simulink model "StraddleCarrier"  (R2022b)
settings: Solver=FixedStepAuto  StartTime=0  StopTime=1000  FixedStep=Ts  RelTol=1e-3
undefined symbols (not defined in the file): AEB, driving, m, n, q, theta, Ts
libraries: simulink x6, roadrunnerscenario x4, simulink_extras x4, drivingscenarioandsensors x3, uavsim3dlib x3, sim3dprobsensorlib x2, trackingutilitieslib x1, drivinglib x1, sim3dlib x1, sim3dcameralib x1, sim3dphyssensorlib x1, sim3dgroundtruthsensorlib x1
(part 2 of 3)

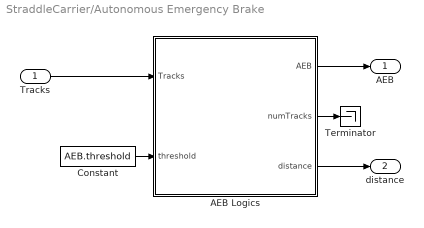
== system StraddleCarrier/Autonomous Emergency Brake ==
  Tracks : Inport  OutDataTypeStr=Bus: BusMultiObjectTracker1  SampleTime=[Ts, 0]  BusOutputAsStruct=on
  AEB Logics : MATLAB Function  TreatAsAtomicUnit=on
  Constant : Constant  Value=AEB.threshold
  Terminator : Terminator
  AEB : Outport  OutDataTypeStr=boolean
  distance : Outport  Port=2
  wires:
  Tracks/1 -> AEB Logics/1(Tracks)
  AEB Logics/1(AEB) -> AEB/1
  Constant/1 -> AEB Logics/2(threshold)
  AEB Logics/3(distance) -> distance/1
  AEB Logics/2(numTracks) -> Terminator/1

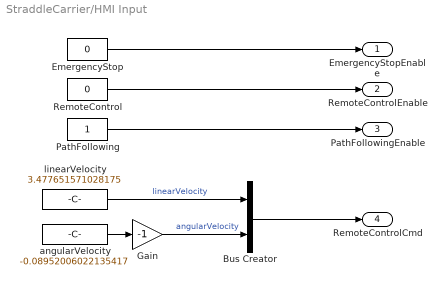
== system StraddleCarrier/HMI Input ==
  Bus Creator : BusCreator  Inputs=2  OutDataTypeStr=Bus: RemoteControlCmd
  EmergencyStop : Constant  Value=0  OutDataTypeStr=boolean
  Gain : Gain  Gain=-1
  PathFollowing : Constant  OutDataTypeStr=boolean
  RemoteControl : Constant  Value=0  OutDataTypeStr=boolean
  angularVelocity : Constant  Value=-0.08952006022135417
  linearVelocity : Constant  Value=3.477651571028175
  EmergencyStopEnable : Outport
  RemoteControlEnable : Outport  Port=2
  PathFollowingEnable : Outport  Port=3
  RemoteControlCmd : Outport  Port=4
  wires:
  RemoteControl/1 -> RemoteControlEnable/1
  linearVelocity/1 -> Bus Creator/1  "linearVelocity"
  PathFollowing/1 -> PathFollowingEnable/1
  angularVelocity/1 -> Gain/1
  EmergencyStop/1 -> EmergencyStopEnable/1
  Bus Creator/1 -> RemoteControlCmd/1
  Gain/1 -> Bus Creator/2  "angularVelocity"

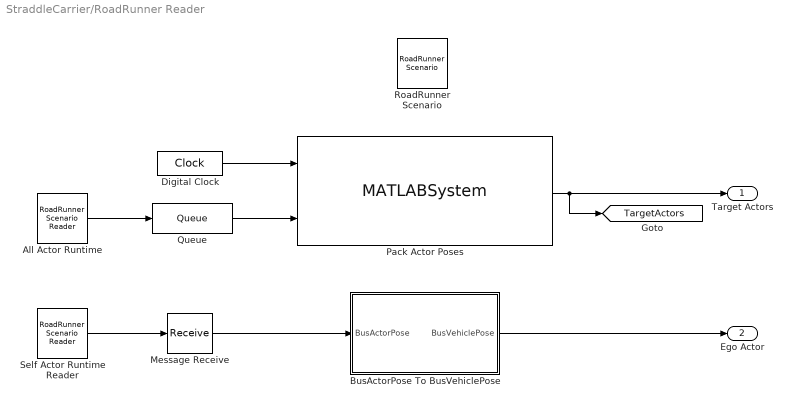
== system StraddleCarrier/RoadRunner Reader ==
  All Actor Runtime : roadrunnerscenario/RoadRunner Scenario Reader  TopicCategory=Actor  ActorCategory=All Types  ActionType=Path Following  TopicType=Actor Pose (Driving Scenario compatible)  VehicleType=Vehicle Specifications  UserDefinedAction=Action1  Filter=None  SampleTime=Ts
  BusActorPose To BusVehiclePose : Subsystem
  Digital Clock : DigitalClock  SampleTime=Ts
  Message Receive : Receive  InputPortMessageModes=m  SampleTime=Ts
  Pack Actor Poses : MATLABSystem  InputPortMessageModes=n,m  System=HelperPackDrivingScenarioPoses  EgoActorID=1  ActorProfiles=struct( 'ActorID', 1, 'ClassID', 1, 'Length', 4.7, 'Width', 1.8, 'Height', 1.4, 'OriginOffset', [ 0, 0, 0 ], 'FrontOverhang', 0, 'RearOverhang', 0, 'Wheelbase', 0, 'Color', [ 0, 0, 0 ] )  DefaultActorPoses="Simulink.Bus.createMATLABStruct( \"BusActors\" )"
      mask Type: HelperPackDrivingScenarioPoses
      mask Display:
      | disp(['HelperPack' char(10) 'DrivingScenarioPoses']);
      | port_label('input',1,'time');
      | port_label('input',2,'msgs');
      | port_label('output',1,'TargetPoses');
  Queue : Queue  InputPortMessageModes=m  OutputPortMessageModes=m  OverwriteOldest=on  Capacity=numActors
  RoadRunner Scenario : roadrunnerscenario/RoadRunner Scenario  UserDefinedActions={}
  Self Actor Runtime Reader : roadrunnerscenario/RoadRunner Scenario Reader  TopicCategory=Actor  ActorCategory=All Types  ActionType=Path Following  TopicType=Actor Pose (Driving Scenario compatible)  VehicleType=Vehicle Specifications  UserDefinedAction=Action1  Filter=Self  SampleTime=Ts
  Target Actors : Outport
  Ego Actor : Outport  Port=2
  tag scope: TargetActors=global
  wires:
  All Actor Runtime/1 -> Queue/1
  Self Actor Runtime Reader/1 -> Message Receive/1
  Queue/1 -> Pack Actor Poses/2
  Pack Actor Poses/1 -> [TargetActors], Target Actors/1
  Message Receive/1 -> BusActorPose To BusVehiclePose/1(BusActorPose)
  BusActorPose To BusVehiclePose/1(BusVehiclePose) -> Ego Actor/1
  Digital Clock/1 -> Pack Actor Poses/1

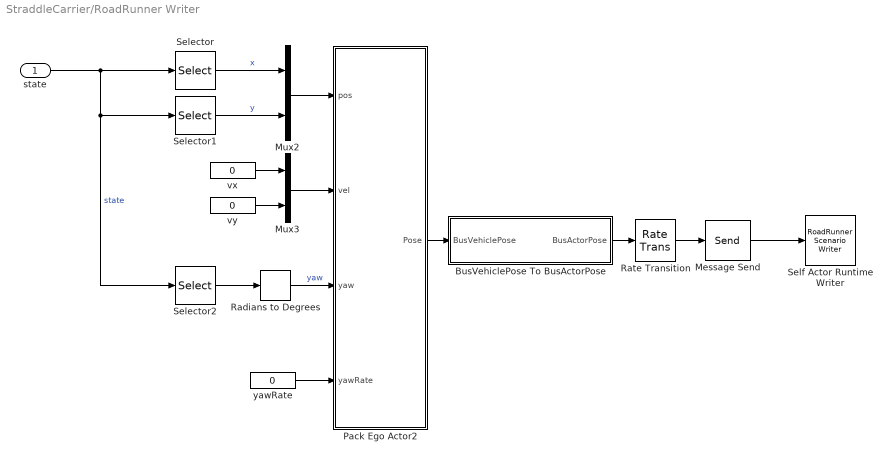
== system StraddleCarrier/RoadRunner Writer ==
  state : Inport
  BusVehiclePose To BusActorPose : Subsystem
  Message Send : Send  OutputPortMessageModes=m
  Mux2 : Mux  Inputs=2
  Mux3 : Mux  Inputs=2
  Pack Ego Actor2 : MATLAB Function  TreatAsAtomicUnit=on  mask{egoActorID=1}
      mask prompts: egoActorID "Ego Actor ID"
  Radians to Degrees : simulink_extras/Transformations/Radians to Degrees
  Rate Transition : RateTransition  OutPortSampleTime=Ts
  Selector : Selector  InputPortWidth=3  IndexOptions=Index vector (dialog)  Indices=[1]  OutputSizes=1
  Selector1 : Selector  InputPortWidth=3  IndexOptions=Index vector (dialog)  Indices=[2]  OutputSizes=1
  Selector2 : Selector  InputPortWidth=3  IndexOptions=Index vector (dialog)  Indices=[3]  OutputSizes=1
  Self Actor Runtime Writer : roadrunnerscenario/RoadRunner Scenario Writer  TopicCategory=Actor  ActorCategory=All Types  EventType=Action Complete  VehicleType=Vehicle Pose  TopicType=Actor Pose (Driving Scenario compatible)
  vx : Constant  Value=0
  vy : Constant  Value=0
  yawRate : Constant  Value=0
  wires:
  BusVehiclePose To BusActorPose/1(BusActorPose) -> Rate Transition/1
  Pack Ego Actor2/1(Pose) -> BusVehiclePose To BusActorPose/1(BusVehiclePose)
  Message Send/1 -> Self Actor Runtime Writer/1
  Rate Transition/1 -> Message Send/1
  Radians to Degrees/1 -> Pack Ego Actor2/3(yaw)  "yaw"
  state/1 -> Selector2/1, Selector1/1, Selector/1  "state"
  vx/1 -> Mux3/1
  vy/1 -> Mux3/2
  Selector1/1 -> Mux2/2  "y"
  Mux3/1 -> Pack Ego Actor2/2(vel)
  Mux2/1 -> Pack Ego Actor2/1(pos)
  Selector/1 -> Mux2/1  "x"
  yawRate/1 -> Pack Ego Actor2/4(yawRate)
  Selector2/1 -> Radians to Degrees/1

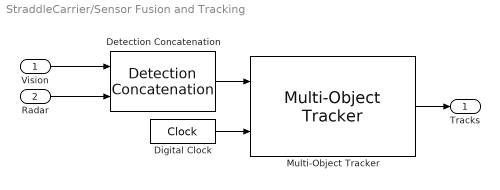
== system StraddleCarrier/Sensor Fusion and Tracking ==
  Vision : Inport  OutDataTypeStr=Bus: BusVision  PortDimensions=[1 1]  SampleTime=[Ts,0]  BusOutputAsStruct=on
  Radar : Inport  Port=2  OutDataTypeStr=Bus: BusRadar  PortDimensions=[1 1]  SampleTime=[Ts,0]  BusOutputAsStruct=on
  Detection Concatenation : trackingutilitieslib/Detection Concatenation  NumInputs=2  BusNameSource=Auto  BusName=BusDetectionConcatenation  SimulateUsing=Code generation
  Digital Clock : DigitalClock  SampleTime=Ts
  Multi-Object Tracker : drivinglib/Multi-Object Tracker  TrackerIndex=uint32( 0 )  FilterInitializationFcn=initcvekf  AssignmentThreshold=50  ConfirmationThreshold=[2, 3]  DeletionThreshold=[3, 3]  MaxNumTracks=20  MaxNumSensors=2  OOSMHandling=Terminate  StateParametersSimulink=struct  HasStateParametersInput=off  TimeInputSource=Input port  HasCostMatrixInput=off  HasDetectableTrackIDsInput=off  BusNameSource=Property  BusName=BusMultiObjectTracker1  TentativeTracksOutputPort=off  AllTracksOutputPort=off  SimulateUsing=Interpreted execution
  Tracks : Outport  OutDataTypeStr=Bus: BusMultiObjectTracker1  PortDimensions=[1 1]  SampleTime=[Ts,0]  VectorParamsAs1DForOutWhenUnconnected=off  BusOutputAsStruct=on
  wires:
  Vision/1 -> Detection Concatenation/1
  Radar/1 -> Detection Concatenation/2
  Detection Concatenation/1 -> Multi-Object Tracker/1
  Multi-Object Tracker/1 -> Tracks/1
  Digital Clock/1 -> Multi-Object Tracker/2

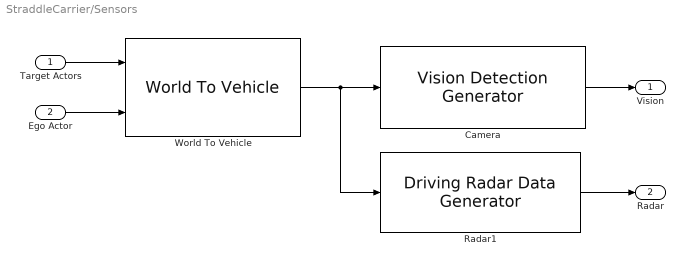
== system StraddleCarrier/Sensors ==
  Target Actors : Inport
  Ego Actor : Inport  Port=2
  Camera : drivingscenarioandsensors/Vision Detection Generator  SensorIndex=1  DetectorOutput=Objects only  UpdateInterval=0.1  LaneUpdateInterval=0.1  SensorLocation=[5 0]  Height=1.1  Yaw=0  Pitch=1  Roll=0  BusNameSource=Auto  BusName=BusObjectDetections  BusName2Source=Auto  BusName2=BusLaneDetections  MaxNumDetectionsSource=Property  MaxNumDetections=20  MaxNumLanesSource=Property  MaxNumLanes=30  DetectionCoordinates=Ego Cartesian  SimulateUsing=Interpreted execution  MaxRange=100  BoundingBoxAccuracy=5  ProcessNoiseIntensity=5  MaxSpeed=100  MaxAllowedOcclusion=0.5  MinObjectImageSize=[15 15]  DetectionProbability=0.9  FalsePositivesPerImage=0.1  MinLaneImageSize=[20 3]  LaneBoundaryAccuracy=3  HasNoise=off  InitialSeedSource=Repeatable  InitialSeed=0  UsedSeed=0  ActorProfilesSource=Parameters  ActorProfilesParameters=driving.internal.ActorProfilesParameters('Length',5,'Width',2,'Height',1.5)  ActorProfilesExpression=[struct('ActorID',1,'ClassID',2,'Length',8.2,'Width',2.5,'Height',3.5,'OriginOffset',[-3.1 0 0],'MeshVertices',[7.2 1.25 1.30597014925373;7.2 -1.25 1.30597014925373;7.2 -1.25 0.574626865671641;7.2 1.25 0.574626865671641;7.2 1.25 1.30597014925373;5.765 1.25 1.67164179104478;5.765 -1.25 1.67164179104478;7.2 -1.25 1.30597014925373;4.945 1 2.58582089552239;4.002 1 2.58582089552239;4.002 -1 2.58582089552239;4.945 -1 2.58582089552239;4.002 1 2.58582089552239;4.002 1.25 1.67164179104478;4.002 -1.25 1.67164179104478;4.002 -1 2.58582089552239;4.002 1.25 1.67164179104478;4.002 1.25 0.574626865671641;4.002 -1.25 0.574626865671641;4.002 -1.25 1.67164179104478;3.92 1.25 3.5;-1 1.25 3.5;-1 -1.25 3.5;3.92 -1.25 3.5;3.92 -1.25 3.5;3.92 -1.25 0.574626865671641;3.92 1.25 0.574626865671641;3.92 1.25 3.5;-1 1.25 3.5;-1 1.25 0.574626865671641;3.92 1.25 0.574626865671641;3.92 1.25 3.5;-1 -1.25 3.5;-1 -1.25 0.574626865671641;3.92 -1.25 0.574626865671641;3.92 -1.25 3.5;5.765 1.25 1.67164179104478;5.355 1.25 1.67164179104478;4.74 1 2.58582089552239;4.945 1 2.58582089552239;7.2 1.25 1.30597014925373;7.2 1.25 0.574626865671641;5.765 1.25 0.574626865671641;5.765 1.25 1.67164179104478;5.765 1.25 1.67164179104478;5.765 1.25 0.574626865671641;4.002 1.25 0.574626865671641;4.002 1.25 1.67164179104478;4.33 1.25 1.67164179104478;4.002 1.25 1.67164179104478;4.002 1 2.58582089552239;4.33 1 2.58582089552239;5.765 -1.25 1.67164179104478;5.355 -1.25 1.67164179104478;4.74 -1 2.58582089552239;4.945 -1 2.58582089552239;7.2 -1.25 1.30597014925373;7.2 -1.25 0.574626865671641;5.765 -1.25 0.574626865671641;5.765 -1.25 1.67164179104478;5.765 -1.25 1.67164179104478;5.765 -1.25 0.574626865671641;4.002 -1.25 0.574626865671641;4.002 -1.25 1.67164179104478;4.33 -1.25 1.67164179104478;4.002 -1.25 1.67164179104478;4.002 -1 2.58582089552239;4.33 -1 2.58582089552239;-1 1.25 3.5;-1 1.25 0.574626865671641;-1 -1.25 0.574626865671641;-1 -1.25 3.5;7.2 1.25 0.574626865671641;7.2 -1.25 0.574626865671641;-1 -1.25 0.574626865671641;-1 1.25 0.574626865671641;0 -0.915 -2.22044604925031e-16;0 -1.185 -2.22044604925031e-16;0.293892626146237 -0.915 0.0997672417444302;0.293892626146237 -1.185 0.0997672417444302;0.475528258147577 -0.915 0.360961271595177;0.475528258147577 -1.185 0.360961271595177;0.475528258147577 -0.915 0.683814847807808;0.475528258147577 -1.185 0.683814847807808;0.293892626146237 -0.915 0.945008877658554;0.293892626146237 -1.185 0.945008877658554;0 -0.915 1.04477611940298;0 -1.185 1.04477611940298;-0.293892626146237 -0.915 0.945008877658554;-0.293892626146237 -1.185 0.945008877658554;-0.475528258147577 -0.915 0.683814847807808;-0.475528258147577 -1.185 0.683814847807808;-0.475528258147577 -0.915 0.360961271595177;-0.475528258147577 -1.185 0.360961271595177;-0.293892626146237 -0.915 0.0997672417444302;-0.293892626146237 -1.185 0.0997672417444302;0 -0.915 -2.22044604925031e-16;0 -1.185 -2.22044604925031e-16;0 -0.915 -2.22044604925031e-16;0.293892626146237 -0.915 0.0997672417444302;0.475528258147577 -0.915 0.360961271595177;0.475528258147577 -0.915 0.683814847807808;0.293892626146237 -0.915 0.945008877658554;0 -0.915 1.04477611940298;-0.293892626146237 -0.915 0.945008877658554;-0.475528258147577 -0.915 0.683814847807808;-0.475528258147577 -0.915 0.360961271595177;-0.293892626146237 -0.915 0.0997672417444302;0 -1.185 -2.22044604925031e-16;0.293892626146237 -1.185 0.0997672417444302;0.475528258147577 -1.185 0.360961271595177;0.475528258147577 -1.185 0.683814847807808;0.293892626146237 -1.185 0.945008877658554;0 -1.185 1.04477611940298;-0.293892626146237 -1.185 0.945008877658554;-0.475528258147577 -1.185 0.683814847807808;-0.475528258147577 -1.185 0.360961271595177;-0.293892626146237 -1.185 0.0997672417444302;0 1.185 -2.22044604925031e-16;0 0.915 -2.22044604925031e-16;0.293892626146237 1.185 0.0997672417444302;0.293892626146237 0.915 0.0997672417444302;0.475528258147577 1.185 0.360961271595177;0.475528258147577 0.915 0.360961271595177;0.475528258147577 1.185 0.683814847807808;0.475528258147577 0.915 0.683814847807808;0.293892626146237 1.185 0.945008877658554;0.293892626146237 0.915 ...(+7888 chars)],'MeshFaces',[1 2 3;3 4 1;5 6 7;7 8 5;9 10 11;11 12 9;13 14 15;15 16 13;17 18 19;19 20 17;21 22 23;23 24 21;25 26 27;27 28 25;29 30 31;31 32 29;33 34 35;35 36 33;37 38 39;39 40 37;41 42 43;43 44 41;45 46 47;47 48 45;49 50 51;51 52 49;53 54 55;55 56 53;57 58 59;59 60 57;61 62 63;63 64 61;65 66 67;67 68 65;69 70 71;71 72 69;73 74 75;75 76 73;77 79 80;80 78 77;79 81 82;82 80 79;81 83 84;84 82 81;83 85 86;86 84 83;85 87 88;88 86 85;87 89 90;90 88 87;89 91 92;92 90 89;91 93 94;94 92 91;93 95 96;96 94 93;95 97 98;98 96 95;99 100 101;99 101 102;99 102 103;99 103 104;99 104 105;99 105 106;99 106 107;99 107 108;109 110 111;109 111 112;109 112 113;109 113 114;109 114 115;109 115 116;109 116 117;109 117 118;119 121 122;122 120 119;121 123 124;124 122 121;123 125 126;126 124 123;125 127 128;128 126 125;127 129 130;130 128 127;129 131 132;132 130 129;131 133 134;134 132 131;133 135 136;136 134 133;135 137 138;138 136 135;137 139 140;140 138 137;141 142 143;141 143 144;141 144 145;141 145 146;141 146 147;141 147 148;141 148 149;141 149 150;151 152 153;151 153 154;151 154 155;151 155 156;151 156 157;151 157 158;151 158 159;151 159 160;161 163 164;164 162 161;163 165 166;166 164 163;165 167 168;168 166 165;167 169 170;170 168 167;169 171 172;172 170 169;171 173 174;174 172 171;173 175 176;176 174 173;175 177 178;178 176 175;177 179 180;180 178 177;179 181 182;182 180 179;183 184 185;183 185 186;183 186 187;183 187 188;183 188 189;183 189 190;183 190 191;183 191 192;193 194 195;193 195 196;193 196 197;193 197 198;193 198 199;193 199 200;193 200 201;193 201 202;203 205 206;206 204 203;205 207 208;208 206 205;207 209 210;210 208 207;209 211 212;212 210 209;211 213 214;214 212 211;213 215 216;216 214 213;215 217 218;218 216 215;217 219 220;220 218 217;219 221 222;222 220 219;221 223 224;224 222 221;225 226 227;225 227 228;225 228 229;225 229 230;225 230 231;225 231 232;225 232 233;225 233 234;235 236 237;235 237 238;235 238 239;235 239 240;235 240 241;235 241 242;235 242 243;235 243 244;245 247 248;248 246 245;247 249 250;250 248 247;249 251 252;252 250 249;251 253 254;254 252 251;253 255 256;256 254 253;255 257 258;258 256 255;257 259 260;260 258 257;259 261 262;262 260 259;261 263 264;264 262 261;263 265 266;266 264 263;267 268 269;267 269 270;267 270 271;267 271 272;267 272 273;267 273 274;267 274 275;267 275 276;277 278 279;277 279 280;277 280 281;277 281 282;277 282 283;277 283 284;277 284 285;277 285 286;287 289 290;290 288 287;289 291 292;292 290 289;291 293 294;294 292 291;293 295 296;296 294 293;295 297 298;298 296 295;297 299 300;300 298 297;299 301 302;302 300 299;301 303 304;304 302 301;303 305 306;306 304 303;305 307 308;308 306 305;309 310 311;309 311 312;309 312 313;309 313 314;309 314 315;309 315 316;309 316 317;309 317 318;319 320 321;319 321 322;319 322 323;319 323 324;319 324 325;319 325 326;319 326 327;319 327 328],'RCSPattern',[10 10;10 10],'RCSAzimuthAngles',[-180 180],'RCSElevationAngles',[-90 90])]  Intrinsics=driving.internal.cameraIntrinsics('FocalLength',[500 500],'PrincipalPoint',[320 240],'ImageSize',[1080 1920],'RadialDistortion',[0 0],'TangentialDistortion',[0 0],'Skew',0)
  Radar1 : drivingscenarioandsensors/Driving Radar Data Generator  SensorIndex=2  UpdateRate=1/Ts  MountingLocation=[5 0 0.2]  MountingAngles=[0 0 0]  HasElevation=on  HasRangeRate=on  HasNoise=off  HasFalseAlarms=off  HasOcclusion=on  MaxNumReportsSource=Property  MaxNumReports=50  TargetReportFormat=Clustered detections  DetectionCoordinates=Body  TrackCoordinates=Body  BusNameSource=Auto  BusName=BusDrivingRadarDataGenerator  AzimuthResolution=2  ElevationResolution=2  RangeResolution=2  RangeRateResolution=0.5  AzimuthBiasFraction=0.1  ElevationBiasFraction=0.1  RangeBiasFraction=0.05  RangeRateBiasFraction=0.05  FieldOfView=[90 5]  RangeLimits=[0 120]  RangeRateLimits=[-100 100]  DetectionProbability=0.9  FalseAlarmRate=1e-06  ReferenceRange=100  ReferenceRCS=0  CenterFrequency=77000000000  FilterInitializationFcn=initcvekf  ConfirmationThreshold=[2 3]  DeletionThreshold=[5 5]  InitialSeedSource=Repeatable  InitialSeed=0  UsedSeed=0  ProfilesSource=Parameters  ProfilesParameters=driving.internal.ActorProfilesRadarParameters('Length',5,'Width',2,'Height',1.5)  ProfilesExpression=[struct('ActorID',1,'ClassID',2,'Length',8.2,'Width',2.5,'Height',3.5,'OriginOffset',[-3.1 0 0],'MeshVertices',[7.2 1.25 1.30597014925373;7.2 -1.25 1.30597014925373;7.2 -1.25 0.574626865671641;7.2 1.25 0.574626865671641;7.2 1.25 1.30597014925373;5.765 1.25 1.67164179104478;5.765 -1.25 1.67164179104478;7.2 -1.25 1.30597014925373;4.945 1 2.58582089552239;4.002 1 2.58582089552239;4.002 -1 2.58582089552239;4.945 -1 2.58582089552239;4.002 1 2.58582089552239;4.002 1.25 1.67164179104478;4.002 -1.25 1.67164179104478;4.002 -1 2.58582089552239;4.002 1.25 1.67164179104478;4.002 1.25 0.574626865671641;4.002 -1.25 0.574626865671641;4.002 -1.25 1.67164179104478;3.92 1.25 3.5;-1 1.25 3.5;-1 -1.25 3.5;3.92 -1.25 3.5;3.92 -1.25 3.5;3.92 -1.25 0.574626865671641;3.92 1.25 0.574626865671641;3.92 1.25 3.5;-1 1.25 3.5;-1 1.25 0.574626865671641;3.92 1.25 0.574626865671641;3.92 1.25 3.5;-1 -1.25 3.5;-1 -1.25 0.574626865671641;3.92 -1.25 0.574626865671641;3.92 -1.25 3.5;5.765 1.25 1.67164179104478;5.355 1.25 1.67164179104478;4.74 1 2.58582089552239;4.945 1 2.58582089552239;7.2 1.25 1.30597014925373;7.2 1.25 0.574626865671641;5.765 1.25 0.574626865671641;5.765 1.25 1.67164179104478;5.765 1.25 1.67164179104478;5.765 1.25 0.574626865671641;4.002 1.25 0.574626865671641;4.002 1.25 1.67164179104478;4.33 1.25 1.67164179104478;4.002 1.25 1.67164179104478;4.002 1 2.58582089552239;4.33 1 2.58582089552239;5.765 -1.25 1.67164179104478;5.355 -1.25 1.67164179104478;4.74 -1 2.58582089552239;4.945 -1 2.58582089552239;7.2 -1.25 1.30597014925373;7.2 -1.25 0.574626865671641;5.765 -1.25 0.574626865671641;5.765 -1.25 1.67164179104478;5.765 -1.25 1.67164179104478;5.765 -1.25 0.574626865671641;4.002 -1.25 0.574626865671641;4.002 -1.25 1.67164179104478;4.33 -1.25 1.67164179104478;4.002 -1.25 1.67164179104478;4.002 -1 2.58582089552239;4.33 -1 2.58582089552239;-1 1.25 3.5;-1 1.25 0.574626865671641;-1 -1.25 0.574626865671641;-1 -1.25 3.5;7.2 1.25 0.574626865671641;7.2 -1.25 0.574626865671641;-1 -1.25 0.574626865671641;-1 1.25 0.574626865671641;0 -0.915 -2.22044604925031e-16;0 -1.185 -2.22044604925031e-16;0.293892626146237 -0.915 0.0997672417444302;0.293892626146237 -1.185 0.0997672417444302;0.475528258147577 -0.915 0.360961271595177;0.475528258147577 -1.185 0.360961271595177;0.475528258147577 -0.915 0.683814847807808;0.475528258147577 -1.185 0.683814847807808;0.293892626146237 -0.915 0.945008877658554;0.293892626146237 -1.185 0.945008877658554;0 -0.915 1.04477611940298;0 -1.185 1.04477611940298;-0.293892626146237 -0.915 0.945008877658554;-0.293892626146237 -1.185 0.945008877658554;-0.475528258147577 -0.915 0.683814847807808;-0.475528258147577 -1.185 0.683814847807808;-0.475528258147577 -0.915 0.360961271595177;-0.475528258147577 -1.185 0.360961271595177;-0.293892626146237 -0.915 0.0997672417444302;-0.293892626146237 -1.185 0.0997672417444302;0 -0.915 -2.22044604925031e-16;0 -1.185 -2.22044604925031e-16;0 -0.915 -2.22044604925031e-16;0.293892626146237 -0.915 0.0997672417444302;0.475528258147577 -0.915 0.360961271595177;0.475528258147577 -0.915 0.683814847807808;0.293892626146237 -0.915 0.945008877658554;0 -0.915 1.04477611940298;-0.293892626146237 -0.915 0.945008877658554;-0.475528258147577 -0.915 0.683814847807808;-0.475528258147577 -0.915 0.360961271595177;-0.293892626146237 -0.915 0.0997672417444302;0 -1.185 -2.22044604925031e-16;0.293892626146237 -1.185 0.0997672417444302;0.475528258147577 -1.185 0.360961271595177;0.475528258147577 -1.185 0.683814847807808;0.293892626146237 -1.185 0.945008877658554;0 -1.185 1.04477611940298;-0.293892626146237 -1.185 0.945008877658554;-0.475528258147577 -1.185 0.683814847807808;-0.475528258147577 -1.185 0.360961271595177;-0.293892626146237 -1.185 0.0997672417444302;0 1.185 -2.22044604925031e-16;0 0.915 -2.22044604925031e-16;0.293892626146237 1.185 0.0997672417444302;0.293892626146237 0.915 0.0997672417444302;0.475528258147577 1.185 0.360961271595177;0.475528258147577 0.915 0.360961271595177;0.475528258147577 1.185 0.683814847807808;0.475528258147577 0.915 0.683814847807808;0.293892626146237 1.185 0.945008877658554;0.293892626146237 0.915 ...(+7888 chars)],'MeshFaces',[1 2 3;3 4 1;5 6 7;7 8 5;9 10 11;11 12 9;13 14 15;15 16 13;17 18 19;19 20 17;21 22 23;23 24 21;25 26 27;27 28 25;29 30 31;31 32 29;33 34 35;35 36 33;37 38 39;39 40 37;41 42 43;43 44 41;45 46 47;47 48 45;49 50 51;51 52 49;53 54 55;55 56 53;57 58 59;59 60 57;61 62 63;63 64 61;65 66 67;67 68 65;69 70 71;71 72 69;73 74 75;75 76 73;77 79 80;80 78 77;79 81 82;82 80 79;81 83 84;84 82 81;83 85 86;86 84 83;85 87 88;88 86 85;87 89 90;90 88 87;89 91 92;92 90 89;91 93 94;94 92 91;93 95 96;96 94 93;95 97 98;98 96 95;99 100 101;99 101 102;99 102 103;99 103 104;99 104 105;99 105 106;99 106 107;99 107 108;109 110 111;109 111 112;109 112 113;109 113 114;109 114 115;109 115 116;109 116 117;109 117 118;119 121 122;122 120 119;121 123 124;124 122 121;123 125 126;126 124 123;125 127 128;128 126 125;127 129 130;130 128 127;129 131 132;132 130 129;131 133 134;134 132 131;133 135 136;136 134 133;135 137 138;138 136 135;137 139 140;140 138 137;141 142 143;141 143 144;141 144 145;141 145 146;141 146 147;141 147 148;141 148 149;141 149 150;151 152 153;151 153 154;151 154 155;151 155 156;151 156 157;151 157 158;151 158 159;151 159 160;161 163 164;164 162 161;163 165 166;166 164 163;165 167 168;168 166 165;167 169 170;170 168 167;169 171 172;172 170 169;171 173 174;174 172 171;173 175 176;176 174 173;175 177 178;178 176 175;177 179 180;180 178 177;179 181 182;182 180 179;183 184 185;183 185 186;183 186 187;183 187 188;183 188 189;183 189 190;183 190 191;183 191 192;193 194 195;193 195 196;193 196 197;193 197 198;193 198 199;193 199 200;193 200 201;193 201 202;203 205 206;206 204 203;205 207 208;208 206 205;207 209 210;210 208 207;209 211 212;212 210 209;211 213 214;214 212 211;213 215 216;216 214 213;215 217 218;218 216 215;217 219 220;220 218 217;219 221 222;222 220 219;221 223 224;224 222 221;225 226 227;225 227 228;225 228 229;225 229 230;225 230 231;225 231 232;225 232 233;225 233 234;235 236 237;235 237 238;235 238 239;235 239 240;235 240 241;235 241 242;235 242 243;235 243 244;245 247 248;248 246 245;247 249 250;250 248 247;249 251 252;252 250 249;251 253 254;254 252 251;253 255 256;256 254 253;255 257 258;258 256 255;257 259 260;260 258 257;259 261 262;262 260 259;261 263 264;264 262 261;263 265 266;266 264 263;267 268 269;267 269 270;267 270 271;267 271 272;267 272 273;267 273 274;267 274 275;267 275 276;277 278 279;277 279 280;277 280 281;277 281 282;277 282 283;277 283 284;277 284 285;277 285 286;287 289 290;290 288 287;289 291 292;292 290 289;291 293 294;294 292 291;293 295 296;296 294 293;295 297 298;298 296 295;297 299 300;300 298 297;299 301 302;302 300 299;301 303 304;304 302 301;303 305 306;306 304 303;305 307 308;308 306 305;309 310 311;309 311 312;309 312 313;309 313 314;309 314 315;309 315 316;309 316 317;309 317 318;319 320 321;319 321 322;319 322 323;319 323 324;319 324 325;319 325 326;319 326 327;319 327 328],'RCSPattern',[10 10;10 10],'RCSAzimuthAngles',[-180 180],'RCSElevationAngles',[-90 90])]
  World To Vehicle : drivingscenarioandsensors/World To Vehicle  BusNameSource=Auto  BusName=BusWorldToVehicleActors  SimulateUsing=Interpreted execution
  Vision : Outport  OutDataTypeStr=Bus: BusVision
  Radar : Outport  Port=2
  wires:
  Ego Actor/1 -> World To Vehicle/2
  World To Vehicle/1 -> Radar1/1, Camera/1
  Target Actors/1 -> World To Vehicle/1
  Radar1/1 -> Radar/1
  Camera/1 -> Vision/1

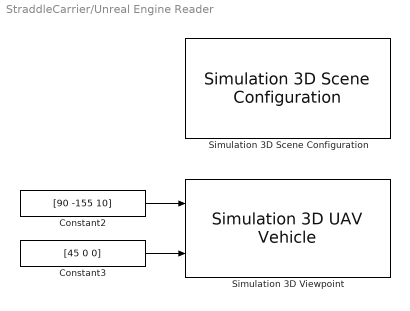
== system StraddleCarrier/Unreal Engine Reader ==
  Constant2 : Constant  Value=[90 -155 10]
  Constant3 : Constant  Value=[45 0 0]
  Simulation 3D Scene Configuration : sim3dlib/Simulation 3D Scene Configuration  Priority=0  ProjectFormat=Unreal Editor  SceneDesc=US city block  ProjectName=C:\Program Files\MATLAB\R2022b\toolbox\shared\sim3d_projects\automotive_project\UE4\WindowsNoEditor\VehicleSimulation.exe  ScenePath=/Game/Maps/USCityBlock  UEProjPath=C:\OffRoad\StraddleCarrier\UnrealEngine\StraddleCarrier\StraddleCarrier.uproject  EnableOpenDRIVE=off  vehTagList={'Scene Origin';'SimulinkVehicle1';'SimulinkVehicleEgo';'SimulinkViewpoint'}  vehTag=SimulinkViewpoint  OpVisEn=off  Ts=Ts  EnableWindow=on  EnableRemoteAccess=off  EnableWeather=off  SunAltitude=40.0  SunAzimuth=90  clouds=10  wind=1  fog=0  rain=0  EnableGeospatial=off  OriginHeight=200  OriginLatitude=40.744652  OriginLongitude=-73.988864  MapStyle=Aerial  AdditionalAssetIDs=[]  UseAdvancedSunSky=off  SolarTime=11  TimeZone=-5  Day=21  Month=9  Year=2022  UseDaylightSavingTime=on  DSTStartDay=10  DSTStartMonth=3  DSTEndDay=3  DSTEndMonth=11  DSTSwitchHour=2  sensorTag=MainCamera1  sensorId=1  sensorName=MainCamera1  mountLoc=Origin  offsetFlag=off  tmountOffset=[0, 0, 0]  rmountOffset=[0, 0, 0]  HorizontalResolution=1280  VerticalResolution=720  HorizontalFOV=60  mountPoint=[0 0 0]  mountOrientation=[0 0 0]  aMode=4  ID=1  GeoTrigger=Inactive
      settings: LibrarySourceBlock=uavsim3dlib/Simulation 3D Scene Configuration
  Simulation 3D Viewpoint : uavsim3dlib/Simulation 3D UAV Vehicle  Priority=-1  Mesh=Custom  MeshPath=/MathWorksUAVContent/UAVs/Custom/Box.Box  Color=Black  ActorName=SimulinkViewpoint  InitialTranslation=[0 0 0]  InitialRotation=[0 0 0]  SampleTime=-1  ActorType=SimulinkVehicle  ID=C  aMode=4  ActorTag=SimulinkViewpoint
  wires:
  Constant3/1 -> Simulation 3D Viewpoint/2
  Constant2/1 -> Simulation 3D Viewpoint/1

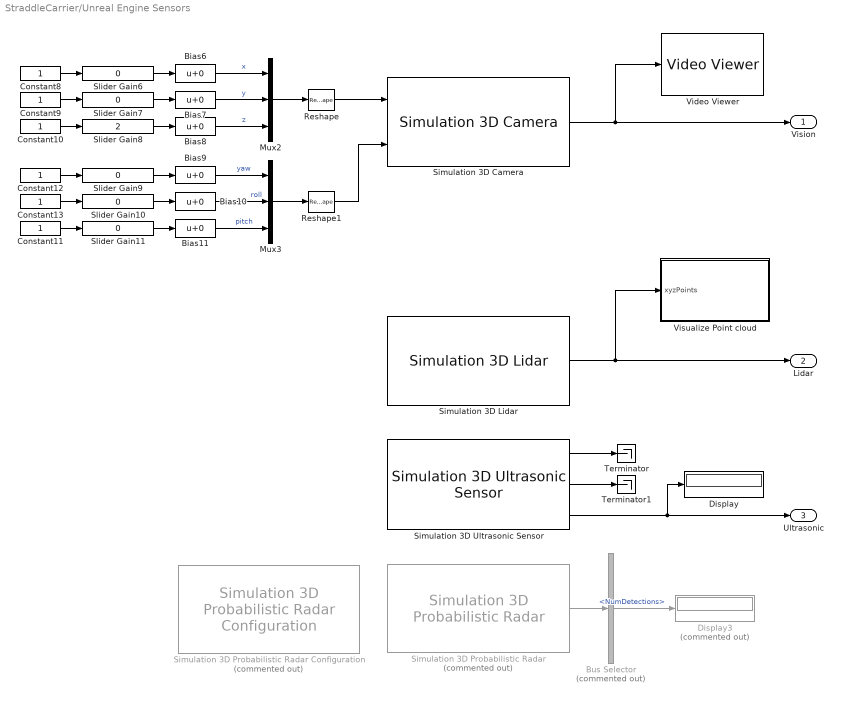
== system StraddleCarrier/Unreal Engine Sensors ==
  Bias{6..11} (6 alike) : Bias  SaturateOnIntegerOverflow=off
  Bus Selector : BusSelector  Commented=on  OutputSignals=NumDetections
  Constant{8..13} (6 alike) : Constant
  Display : Display
  Display3 : Display  Commented=on
  Mux2 : Mux  Inputs=3
  Mux3 : Mux  Inputs=3
  Reshape : Reshape  OutputDimensionality=Customize  OutputDimensions=[1,3]
  Reshape1 : Reshape  OutputDimensionality=Customize  OutputDimensions=[1,3]
  Simulation 3D Camera : sim3dcameralib/Simulation 3D Camera  Priority=1  sensorTag=Sim3dSensor1  sensorId=1  sensorName=Sim3dSensor1  vehTagList={'Scene Origin';'SimulinkVehicle1';'SimulinkVehicleEgo';'SimulinkViewpoint'}  vehTag=SimulinkVehicleEgo  mountLoc=Origin  offsetFlag=on  tmountOffset=[2, 0, 1]  extTmount=on  rmountOffset=[0, 0, 90]  extRmount=on  FocalLength=[1109, 1109]  OpticalCenter=[640, 360]  ImageSize=[720, 1280]  RadialDistortion=[0, 0]  TangentialDistortion=[0, 0]  SensorSkew=0  DepthOutportEnabled=off  SemanticOutportEnabled=off  TransformOutportEnabled=off  SampleTime=-1  mountPoint=[2 0 1]  mountOrientation=[0 0 -90]  aMode=4  ID=1
      settings: LibrarySourceBlock=uavsim3dlib/Simulation 3D Camera
  Simulation 3D Lidar : sim3dphyssensorlib/Simulation 3D Lidar  Priority=1  sensorTag=Sim3dSensor2  sensorId=2  sensorName=Sim3dSensor2  vehTagList={'Scene Origin';'SimulinkVehicleEgo';'SimulinkViewpoint'}  vehTag=SimulinkVehicleEgo  mountLoc=Origin  offsetFlag=on  tmountOffset=[0, 20, 3]  rmountOffset=[0, 0, 90]  DetectionRange=300  RangeResolution=0.002  VerticalFOV=40  VerticalResolution=1.25  HorizontalFOV=360  HorizontalResolution=0.16  DistanceOutportEnabled=off  ReflectivityOutportEnabled=off  SemanticOutportEnabled=off  TransformOutportEnabled=off  SampleTime=-1  mountPoint=[0 -20 3]  mountOrientation=[0 0 -90]  aMode=4  ID=2
      settings: LibrarySourceBlock=uavsim3dlib/Simulation 3D Lidar
  Simulation 3D Probabilistic Radar : sim3dprobsensorlib/Simulation 3D Probabilistic Radar  Priority=1  Commented=on  sensorTag=Sim3dSensor3  sensorId=3  sensorName=Sim3dSensor3  vehTagList={'Scene Origin';'SimulinkBox';'SimulinkVehicleEgo'}  vehTag=SimulinkVehicleEgo  mountLoc=Origin  offsetFlag=on  tmountOffset=[0, 0, 2]  rmountOffset=[0, 0, 0]  AzimuthResolution=1  ElevationResolution=1  RangeResolution=1  RangeRateResolution=0.5  AzimuthBiasFraction=0.1  ElevationBiasFraction=0.1  RangeBiasFraction=0.05  RangeRateBiasFraction=0.05  FieldOfView=[30, 5 ]  DetectionRange=[0.01, 150 ]  RangeRateLimits=[ -100, 100 ]  DetectionProbability=0.9  FalseAlarmRate=1e-6  ReferenceRange=150  ReferenceRCS=0  HasElevation=on  HasRangeRate=on  HasNoise=off  HasFalseAlarms=off  InitialSeedSource=Repeatable  InitialSeed=0  MaxNumDetections=10  DetectionCoordinates=Ego Cartesian  SpecifyOutputBusName=off  BusName=BusSimulation3DRadarTruthSensor  SampleTime=Ts  mountPoint=[0 0 2]  mountOrientation=[0 0 0]  aMode=3  ID=3
      settings: LibrarySourceBlock=drivingsim3d/Simulation 3D Probabilistic Radar
  Simulation 3D Probabilistic Radar Configuration : sim3dprobsensorlib/Simulation 3D Probabilistic Radar Configuration  Commented=on  RCSactorKeys=[10]  RCSactorProfiles={[10, 10;10, 10]}  RCSdefaultValue=-20  aMode=3
  Simulation 3D Ultrasonic Sensor : sim3dgroundtruthsensorlib/Simulation 3D Ultrasonic Sensor  Priority=1  sensorTag=Sim3dSensor4  sensorId=4  sensorName=Sim3dSensor4  vehTagList={'Scene Origin';'SimulinkVehicle1';'SimulinkVehicleEgo';'SimulinkViewpoint'}  vehTag=SimulinkVehicleEgo  mountLoc=Origin  offsetFlag=on  tmountOffset=[0, 0, 2]  rmountOffset=[0, 0, 90]  detectionRanges=[0.01 0.5 200]  HorizontalFoV=10  VerticalFoV=10  useBusOutput=off  SampleTime=-1  mountPoint=[0 0 2]  mountOrientation=[0 0 -90]  aMode=3  ID=4
      settings: LibrarySourceBlock=drivingsim3d/Simulation 3D Ultrasonic Sensor
  Slider Gain10 : simulink/Math Operations/Slider Gain  gain=0  low=-45  high=45
  Slider Gain11 : simulink/Math Operations/Slider Gain  gain=0  low=-45  high=45
  Slider Gain6 : simulink/Math Operations/Slider Gain  gain=0  low=-5  high=5
  Slider Gain7 : simulink/Math Operations/Slider Gain  gain=0  low=-5  high=5
  Slider Gain8 : simulink/Math Operations/Slider Gain  gain=2  low=-5  high=5
  Slider Gain9 : simulink/Math Operations/Slider Gain  gain=0  low=-45  high=45
  Terminator : Terminator
  Terminator1 : Terminator
  Video Viewer : VideoViewer  FigPos=[605 1001 1284 760]
  Visualize Point cloud : MATLAB Function  StopFcn=|  TreatAsAtomicUnit=on
      | playerFigure = findall(groot,'type','figure','name','Point Cloud Player');
      | 
      | if ~isempty(playerFigure)
      |     playerFigure = playerFigure(end);
      |     if isvalid(playerFigure)
      |         close(playerFigure);
      |     end
      | end
  Vision : Outport
  Lidar : Outport  Port=2
  Ultrasonic : Outport  Port=3
  wires:
  Slider Gain11/1 -> Bias11/1
  Reshape1/1 -> Simulation 3D Camera/2
  Bias11/1 -> Mux3/3  "pitch"
  Slider Gain9/1 -> Bias9/1
  Slider Gain10/1 -> Bias10/1
  Constant13/1 -> Slider Gain10/1
  Bias9/1 -> Mux3/1  "yaw"
  Constant9/1 -> Slider Gain7/1
  Mux2/1 -> Reshape/1
  Bias6/1 -> Mux2/1  "x"
  Bias10/1 -> Mux3/2  "roll"
  Bias7/1 -> Mux2/2  "y"
  Constant12/1 -> Slider Gain9/1
  Mux3/1 -> Reshape1/1
  Bias8/1 -> Mux2/3  "z"
  Constant11/1 -> Slider Gain11/1
  Slider Gain7/1 -> Bias7/1
  Bus Selector/1 -> Display3/1  "<NumDetections>"
  Slider Gain6/1 -> Bias6/1
  Slider Gain8/1 -> Bias8/1
  Reshape/1 -> Simulation 3D Camera/1
  Constant10/1 -> Slider Gain8/1
  Simulation 3D Probabilistic Radar/1 -> Bus Selector/1
  Constant8/1 -> Slider Gain6/1
  Simulation 3D Lidar/1 -> Lidar/1, Visualize Point cloud/1(xyzPoints)
  Simulation 3D Camera/1 -> Vision/1, Video Viewer/1
  Simulation 3D Ultrasonic Sensor/1 -> Terminator/1
  Simulation 3D Ultrasonic Sensor/2 -> Terminator1/1
  Simulation 3D Ultrasonic Sensor/3 -> Display/1, Ultrasonic/1

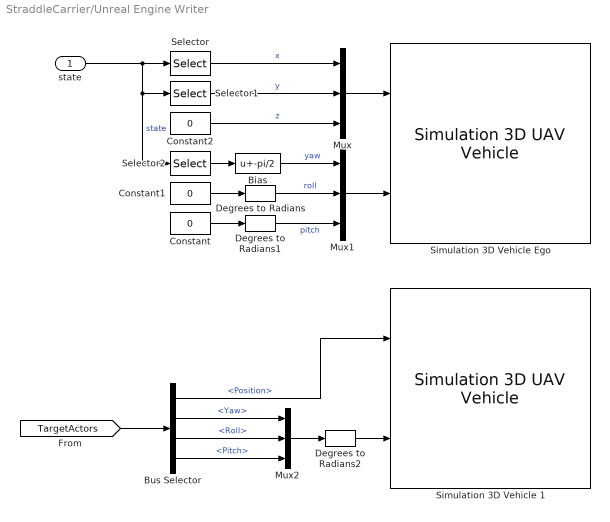
== system StraddleCarrier/Unreal Engine Writer ==
  state : Inport
  Bias : Bias  Bias=-pi/2  SaturateOnIntegerOverflow=off
  Bus Selector : BusSelector  OutputSignals=Actors.Position,Actors.Yaw,Actors.Roll,Actors.Pitch
  Constant : Constant  Value=0
  Constant1 : Constant  Value=0
  Constant2 : Constant  Value=0
  Degrees to Radians : simulink_extras/Transformations/Degrees to Radians
  Degrees to Radians1 : simulink_extras/Transformations/Degrees to Radians
  Degrees to Radians2 : simulink_extras/Transformations/Degrees to Radians
  Mux : Mux  Inputs=3
  Mux1 : Mux  Inputs=3
  Mux2 : Mux  Inputs=3
  Selector : Selector  InputPortWidth=3  IndexOptions=Index vector (dialog)  Indices=[1]  OutputSizes=1
  Selector1 : Selector  InputPortWidth=3  IndexOptions=Index vector (dialog)  Indices=[2]  OutputSizes=1
  Selector2 : Selector  InputPortWidth=3  IndexOptions=Index vector (dialog)  Indices=[3]  OutputSizes=1
  Simulation 3D Vehicle 1 : uavsim3dlib/Simulation 3D UAV Vehicle  Priority=-1  Mesh=Custom  MeshPath=/MathWorksUAVContent/UAVs/Custom/AmbulanceRed.AmbulanceRed  Color=Black  ActorName=SimulinkVehicle1  InitialTranslation=[0 0 0]  InitialRotation=[0 0 0]  SampleTime=-1  ActorType=SimulinkVehicle  ID=1  aMode=4  ActorTag=SimulinkVehicle1
  Simulation 3D Vehicle Ego : uavsim3dlib/Simulation 3D UAV Vehicle  Priority=-1  Mesh=Custom  MeshPath=/MathWorksUAVContent/UAVs/Custom/Strad_UAV.Strad_UAV  Color=Black  ActorName=SimulinkVehicleEgo  InitialTranslation=[0 0 0]  InitialRotation=[0 0 0]  SampleTime=-1  ActorType=SimulinkVehicle  ID=C  aMode=4  ActorTag=SimulinkVehicleEgo
  wires:
  Selector2/1 -> Bias/1
  Mux/1 -> Simulation 3D Vehicle Ego/1
  Constant2/1 -> Mux/3  "z"
  Mux1/1 -> Simulation 3D Vehicle Ego/2
  Constant/1 -> Degrees to Radians1/1
  Constant1/1 -> Degrees to Radians/1
  Selector1/1 -> Mux/2  "y"
  Selector/1 -> Mux/1  "x"
  state/1 -> Selector/1, Selector2/1, Selector1/1  "state"
  Degrees to Radians/1 -> Mux1/2  "roll"
  Degrees to Radians1/1 -> Mux1/3  "pitch"
  Bias/1 -> Mux1/1  "yaw"
  Bus Selector/1 -> Simulation 3D Vehicle 1/1  "<Position>"
  [TargetActors] -> Bus Selector/1
  Mux2/1 -> Degrees to Radians2/1
  Bus Selector/2 -> Mux2/1  "<Yaw>"
  Bus Selector/3 -> Mux2/2  "<Roll>"
  Bus Selector/4 -> Mux2/3  "<Pitch>"
  Degrees to Radians2/1 -> Simulation 3D Vehicle 1/2
